simulink model "IEEE14_case"  (R2024b)
settings: Solver=FixedStepAuto  StartTime=0  StopTime=2  FixedStep=1e-7  RelTol=1e-3
values from neighbouring files (symbols this model uses):
  GFL_15_Bva = 0.009    [IEEE14_parameters.m]
  GFL_15_C_bus_pu = 7.179419    [IEEE14_parameters.m]
  GFL_15_f0 = 60    [IEEE14_parameters.m]
  GFL_15_I_id = 691.26967    [IEEE14_parameters.m]
  GFL_15_I_iq = 691.26967    [IEEE14_parameters.m]
  GFL_15_I_od = 45.2207    [IEEE14_parameters.m]
  GFL_15_I_oq = 45.2207    [IEEE14_parameters.m]
  GFL_15_I_pll = 0.78    [IEEE14_parameters.m]
  GFL_15_Kdi = 0.09    [IEEE14_parameters.m]
  GFL_15_Kdo = 0.9    [IEEE14_parameters.m]
  GFL_15_Kqi = 0.09    [IEEE14_parameters.m]
  GFL_15_Kqo = 0.9    [IEEE14_parameters.m]
  GFL_15_Lg_pu = 0.631447    [IEEE14_parameters.m]
  GFL_15_mode = 1    [IEEE14_parameters.m]
  GFL_15_P_id = 3.7166    [IEEE14_parameters.m]
  GFL_15_P_iq = 3.7166    [IEEE14_parameters.m]
  GFL_15_P_od = 0.4798    [IEEE14_parameters.m]
  GFL_15_P_oq = 0.4798    [IEEE14_parameters.m]
  GFL_15_P_pll = 290.42    [IEEE14_parameters.m]
  GFL_15_Qe_ref = 0.2    [IEEE14_parameters.m]
  GFL_15_Rg_pu = 0.024016    [IEEE14_parameters.m]
  GFL_15_Sbase = 1.000000e+4    (= 10000)    [IEEE14_parameters.m]
  GFL_15_Tdi = 0.01    [IEEE14_parameters.m]
  GFL_15_Tdo = 0.2    [IEEE14_parameters.m]
  GFL_15_Tqi = 0.01    [IEEE14_parameters.m]
  GFL_15_Tqo = 0.2    [IEEE14_parameters.m]
  GFL_15_Vbase = 380    [IEEE14_parameters.m]
  GFL_15_Vdc_ref = 1.011475    [IEEE14_parameters.m]
  GFL_15_Vdcbase = 700    [IEEE14_parameters.m]
  GFL_15_vq_ref = 0    [IEEE14_parameters.m]
  GFL_16_Bva = 0.002    [IEEE14_parameters.m]
  GFL_16_C_bus_pu = 7.179419    [IEEE14_parameters.m]
  GFL_16_f0 = 60    [IEEE14_parameters.m]
  GFL_16_I_id = 691.26967    [IEEE14_parameters.m]
  GFL_16_I_iq = 691.26967    [IEEE14_parameters.m]
  GFL_16_I_od = 45.2207    [IEEE14_parameters.m]
  GFL_16_I_oq = 45.2207    [IEEE14_parameters.m]
  GFL_16_I_pll = 0.78    [IEEE14_parameters.m]
  GFL_16_Kdi = 0.05    [IEEE14_parameters.m]
  GFL_16_Kdo = 0.5    [IEEE14_parameters.m]
  GFL_16_Kqi = 0.05    [IEEE14_parameters.m]
  GFL_16_Kqo = 0.5    [IEEE14_parameters.m]
  GFL_16_Lg_pu = 0.631447    [IEEE14_parameters.m]
  GFL_16_mode = 1    [IEEE14_parameters.m]
  GFL_16_P_id = 3.7166    [IEEE14_parameters.m]
  GFL_16_P_iq = 3.7166    [IEEE14_parameters.m]
  GFL_16_P_od = 0.4798    [IEEE14_parameters.m]
  GFL_16_P_oq = 0.4798    [IEEE14_parameters.m]
  GFL_16_P_pll = 290.42    [IEEE14_parameters.m]
  GFL_16_Qe_ref = 0.2    [IEEE14_parameters.m]
  GFL_16_Rg_pu = 0.024016    [IEEE14_parameters.m]
  GFL_16_Sbase = 1.000000e+4    (= 10000)    [IEEE14_parameters.m]
  GFL_16_Tdi = 0.01    [IEEE14_parameters.m]
  GFL_16_Tdo = 0.2    [IEEE14_parameters.m]
  GFL_16_Tqi = 0.01    [IEEE14_parameters.m]
  GFL_16_Tqo = 0.2    [IEEE14_parameters.m]
  GFL_16_Vbase = 380    [IEEE14_parameters.m]
  GFL_16_Vdc_ref = 1.01144    [IEEE14_parameters.m]
  GFL_16_Vdcbase = 700    [IEEE14_parameters.m]
  GFL_16_vq_ref = 0    [IEEE14_parameters.m]
  GFL_17_Bva = 0.002    [IEEE14_parameters.m]
  GFL_17_C_bus_pu = 7.179419    [IEEE14_parameters.m]
  GFL_17_f0 = 60    [IEEE14_parameters.m]
  GFL_17_I_id = 691.26967    [IEEE14_parameters.m]
  GFL_17_I_iq = 691.26967    [IEEE14_parameters.m]
  GFL_17_I_od = 45.2207    [IEEE14_parameters.m]
  GFL_17_I_oq = 45.2207    [IEEE14_parameters.m]
  GFL_17_I_pll = 0.78    [IEEE14_parameters.m]
  GFL_17_Kdi = 0.05    [IEEE14_parameters.m]
  GFL_17_Kdo = 0.5    [IEEE14_parameters.m]
  GFL_17_Kqi = 0.05    [IEEE14_parameters.m]
  GFL_17_Kqo = 0.5    [IEEE14_parameters.m]
  GFL_17_Lg_pu = 0.631447    [IEEE14_parameters.m]
  GFL_17_mode = 1    [IEEE14_parameters.m]
  GFL_17_P_id = 3.7166    [IEEE14_parameters.m]
  GFL_17_P_iq = 3.7166    [IEEE14_parameters.m]
  GFL_17_P_od = 0.4798    [IEEE14_parameters.m]
  GFL_17_P_oq = 0.4798    [IEEE14_parameters.m]
  GFL_17_P_pll = 290.42    [IEEE14_parameters.m]
  GFL_17_Qe_ref = 0.2    [IEEE14_parameters.m]
  GFL_17_Rg_pu = 0.024016    [IEEE14_parameters.m]
  GFL_17_Sbase = 1.000000e+4    (= 10000)    [IEEE14_parameters.m]
  GFL_17_Tdi = 0.01    [IEEE14_parameters.m]
  GFL_17_Tdo = 0.2    [IEEE14_parameters.m]
  GFL_17_Tqi = 0.01    [IEEE14_parameters.m]
  GFL_17_Tqo = 0.2    [IEEE14_parameters.m]
  GFL_17_Vbase = 380    [IEEE14_parameters.m]
  GFL_17_Vdc_ref = 1.011632    [IEEE14_parameters.m]
  GFL_17_Vdcbase = 700    [IEEE14_parameters.m]
  GFL_17_vq_ref = 0    [IEEE14_parameters.m]
  GFL_18_Bva = 0.002    [IEEE14_parameters.m]
  GFL_18_C_bus_pu = 7.179419    [IEEE14_parameters.m]
  GFL_18_f0 = 60    [IEEE14_parameters.m]
  GFL_18_I_id = 691.26967    [IEEE14_parameters.m]
  GFL_18_I_iq = 691.26967    [IEEE14_parameters.m]
  GFL_18_I_od = 45.2207    [IEEE14_parameters.m]
  GFL_18_I_oq = 45.2207    [IEEE14_parameters.m]
  GFL_18_I_pll = 0.78    [IEEE14_parameters.m]
  GFL_18_Kdi = 0.05    [IEEE14_parameters.m]
  GFL_18_Kdo = 0.5    [IEEE14_parameters.m]
  GFL_18_Kqi = 0.05    [IEEE14_parameters.m]
  GFL_18_Kqo = 0.5    [IEEE14_parameters.m]
  GFL_18_Lg_pu = 0.631447    [IEEE14_parameters.m]
  GFL_18_mode = 1    [IEEE14_parameters.m]
  GFL_18_P_id = 3.7166    [IEEE14_parameters.m]
  GFL_18_P_iq = 3.7166    [IEEE14_parameters.m]
  GFL_18_P_od = 0.4798    [IEEE14_parameters.m]
  GFL_18_P_oq = 0.4798    [IEEE14_parameters.m]
  GFL_18_P_pll = 290.42    [IEEE14_parameters.m]
  GFL_18_Qe_ref = 0.2    [IEEE14_parameters.m]
  GFL_18_Rg_pu = 0.024016    [IEEE14_parameters.m]
  GFL_18_Sbase = 1.000000e+4    (= 10000)    [IEEE14_parameters.m]
  GFL_18_Tdi = 0.01    [IEEE14_parameters.m]
  GFL_18_Tdo = 0.2    [IEEE14_parameters.m]
  GFL_18_Tqi = 0.01    [IEEE14_parameters.m]
  GFL_18_Tqo = 0.2    [IEEE14_parameters.m]
  GFL_18_Vbase = 380    [IEEE14_parameters.m]
  GFL_18_Vdc_ref = 1.011572    [IEEE14_parameters.m]
  GFL_18_Vdcbase = 700    [IEEE14_parameters.m]
  GFL_18_vq_ref = 0    [IEEE14_parameters.m]
  ... (+180 more)
(part 8 of 25)

== system IEEE14_case/AC_1/d_vq_bus_11_block ==
  note: d_vq_bus_11 in case14gfl
      | $9002.98797417909\,\mathrm{iq}_{\mathrm{bus},11}-376.991118430775\,\mathrm{vd}_{\mathrm{bus},11}$
      | Automatically generated on 2025-10-09 21:38:38 .
  Alge_iq_bus_11_f813e : Inport
  State_vd_bus_11_1dc97 : Inport  Port=2
  Constant_376.991118430775_261c0 : Constant  Value=376.991118430775
  Constant_9002.98797417909_ad544 : Constant  Value=9002.98797417909
  Product_24dc8 : Product
  Product_f14d9 : Product
  Subtract_a07b7 : Sum  Inputs=+-
  Blockout_d_vq_bus_11_d741b : Outport
  wires:
  Constant_9002.98797417909_ad544/1 -> Product_24dc8/1
  Alge_iq_bus_11_f813e/1 -> Product_24dc8/2
  Product_f14d9/1 -> Subtract_a07b7/2
  Constant_376.991118430775_261c0/1 -> Product_f14d9/1
  State_vd_bus_11_1dc97/1 -> Product_f14d9/2
  Product_24dc8/1 -> Subtract_a07b7/1
  Subtract_a07b7/1 -> Blockout_d_vq_bus_11_d741b/1

== system IEEE14_case/AC_1/d_vq_bus_12_block ==
  note: d_vq_bus_12 in case14gfl
      | $3672.44450708959\,\mathrm{iq}_{\mathrm{bus},12}-376.991118430775\,\mathrm{vd}_{\mathrm{bus},12}$
      | Automatically generated on 2025-10-09 21:38:40 .
  Alge_iq_bus_12_a824a : Inport
  State_vd_bus_12_1eb7a : Inport  Port=2
  Constant_3672.44450708959_5aba3 : Constant  Value=3672.44450708959
  Constant_376.991118430775_dbbc3 : Constant  Value=376.991118430775
  Product_f5227 : Product
  Product_ffd2a : Product
  Subtract_7b375 : Sum  Inputs=+-
  Blockout_d_vq_bus_12_08cfc : Outport
  wires:
  Subtract_7b375/1 -> Blockout_d_vq_bus_12_08cfc/1
  Constant_3672.44450708959_5aba3/1 -> Product_f5227/1
  State_vd_bus_12_1eb7a/1 -> Product_ffd2a/2
  Alge_iq_bus_12_a824a/1 -> Product_f5227/2
  Product_ffd2a/1 -> Subtract_7b375/2
  Constant_376.991118430775_dbbc3/1 -> Product_ffd2a/1
  Product_f5227/1 -> Subtract_7b375/1

== system IEEE14_case/AC_1/d_vq_bus_13_block ==
  note: d_vq_bus_13 in case14gfl
      | $2548.2341972351\,\mathrm{iq}_{\mathrm{bus},13}-376.991118430775\,\mathrm{vd}_{\mathrm{bus},13}$
      | Automatically generated on 2025-10-09 21:38:41 .
  Alge_iq_bus_13_d5ed4 : Inport
  State_vd_bus_13_68df6 : Inport  Port=2
  Constant_2548.2341972351_9e862 : Constant  Value=2548.2341972351
  Constant_376.991118430775_4e35a : Constant  Value=376.991118430775
  Product_0bf36 : Product
  Product_4bdfd : Product
  Subtract_14057 : Sum  Inputs=+-
  Blockout_d_vq_bus_13_eb8c6 : Outport
  wires:
  Subtract_14057/1 -> Blockout_d_vq_bus_13_eb8c6/1
  Constant_2548.2341972351_9e862/1 -> Product_0bf36/1
  Alge_iq_bus_13_d5ed4/1 -> Product_0bf36/2
  Constant_376.991118430775_4e35a/1 -> Product_4bdfd/1
  Product_0bf36/1 -> Subtract_14057/1
  State_vd_bus_13_68df6/1 -> Product_4bdfd/2
  Product_4bdfd/1 -> Subtract_14057/2

== system IEEE14_case/AC_1/d_vq_bus_14_block ==
  note: d_vq_bus_14 in case14gfl
      | $20061.7254996805\,\mathrm{iq}_{\mathrm{bus},14}-376.991118430775\,\mathrm{vd}_{\mathrm{bus},14}$
      | Automatically generated on 2025-10-09 21:38:43 .
  Alge_iq_bus_14_0b3bc : Inport
  State_vd_bus_14_b82c6 : Inport  Port=2
  Constant_20061.7254996805_caef0 : Constant  Value=20061.7254996805
  Constant_376.991118430775_d7d60 : Constant  Value=376.991118430775
  Product_cdac7 : Product
  Product_f9a80 : Product
  Subtract_506d5 : Sum  Inputs=+-
  Blockout_d_vq_bus_14_55ab8 : Outport
  wires:
  Constant_20061.7254996805_caef0/1 -> Product_f9a80/1
  Alge_iq_bus_14_0b3bc/1 -> Product_f9a80/2
  Product_cdac7/1 -> Subtract_506d5/2
  State_vd_bus_14_b82c6/1 -> Product_cdac7/2
  Constant_376.991118430775_d7d60/1 -> Product_cdac7/1
  Product_f9a80/1 -> Subtract_506d5/1
  Subtract_506d5/1 -> Blockout_d_vq_bus_14_55ab8/1

== system IEEE14_case/AC_1/d_vq_bus_15_block ==
  note: d_vq_bus_15 in case14gfl
      | $37699.1118430775\,\mathrm{iq}_{\mathrm{bus},15}-376.991118430775\,\mathrm{vd}_{\mathrm{bus},15}$
      | Automatically generated on 2025-10-09 21:38:44 .
  Alge_iq_bus_15_82ed5 : Inport
  State_vd_bus_15_ac75c : Inport  Port=2
  Constant_376.991118430775_eac41 : Constant  Value=376.991118430775
  Constant_37699.1118430775_013c4 : Constant  Value=37699.1118430775
  Product_6e790 : Product
  Product_7bd8f : Product
  Subtract_6bedb : Sum  Inputs=+-
  Blockout_d_vq_bus_15_3c6af : Outport
  wires:
  Constant_37699.1118430775_013c4/1 -> Product_7bd8f/1
  Product_6e790/1 -> Subtract_6bedb/2
  Constant_376.991118430775_eac41/1 -> Product_6e790/1
  Alge_iq_bus_15_82ed5/1 -> Product_7bd8f/2
  State_vd_bus_15_ac75c/1 -> Product_6e790/2
  Product_7bd8f/1 -> Subtract_6bedb/1
  Subtract_6bedb/1 -> Blockout_d_vq_bus_15_3c6af/1

== system IEEE14_case/AC_1/d_vq_bus_16_block ==
  note: d_vq_bus_16 in case14gfl
      | $37699.1118430775\,\mathrm{iq}_{\mathrm{bus},16}-376.991118430775\,\mathrm{vd}_{\mathrm{bus},16}$
      | Automatically generated on 2025-10-09 21:38:46 .
  Alge_iq_bus_16_45d99 : Inport
  State_vd_bus_16_358d8 : Inport  Port=2
  Constant_376.991118430775_caa10 : Constant  Value=376.991118430775
  Constant_37699.1118430775_2a605 : Constant  Value=37699.1118430775
  Product_3e245 : Product
  Product_65d14 : Product
  Subtract_b7523 : Sum  Inputs=+-
  Blockout_d_vq_bus_16_4b2eb : Outport
  wires:
  Alge_iq_bus_16_45d99/1 -> Product_65d14/2
  Constant_37699.1118430775_2a605/1 -> Product_65d14/1
  Product_3e245/1 -> Subtract_b7523/2
  Constant_376.991118430775_caa10/1 -> Product_3e245/1
  State_vd_bus_16_358d8/1 -> Product_3e245/2
  Product_65d14/1 -> Subtract_b7523/1
  Subtract_b7523/1 -> Blockout_d_vq_bus_16_4b2eb/1

== system IEEE14_case/AC_1/d_vq_bus_17_block ==
  note: d_vq_bus_17 in case14gfl
      | $37699.1118430775\,\mathrm{iq}_{\mathrm{bus},17}-376.991118430775\,\mathrm{vd}_{\mathrm{bus},17}$
      | Automatically generated on 2025-10-09 21:38:47 .
  Alge_iq_bus_17_e020e : Inport
  State_vd_bus_17_c4074 : Inport  Port=2
  Constant_376.991118430775_1fb98 : Constant  Value=376.991118430775
  Constant_37699.1118430775_26579 : Constant  Value=37699.1118430775
  Product_819ff : Product
  Product_cf9da : Product
  Subtract_66b2c : Sum  Inputs=+-
  Blockout_d_vq_bus_17_6d857 : Outport
  wires:
  Subtract_66b2c/1 -> Blockout_d_vq_bus_17_6d857/1
  Constant_37699.1118430775_26579/1 -> Product_cf9da/1
  Alge_iq_bus_17_e020e/1 -> Product_cf9da/2
  Constant_376.991118430775_1fb98/1 -> Product_819ff/1
  Product_cf9da/1 -> Subtract_66b2c/1
  State_vd_bus_17_c4074/1 -> Product_819ff/2
  Product_819ff/1 -> Subtract_66b2c/2

== system IEEE14_case/AC_1/d_vq_bus_18_block ==
  note: d_vq_bus_18 in case14gfl
      | $37699.1118430775\,\mathrm{iq}_{\mathrm{bus},18}-376.991118430775\,\mathrm{vd}_{\mathrm{bus},18}$
      | Automatically generated on 2025-10-09 21:38:49 .
  Alge_iq_bus_18_569e7 : Inport
  State_vd_bus_18_940ad : Inport  Port=2
  Constant_376.991118430775_f629c : Constant  Value=376.991118430775
  Constant_37699.1118430775_4526d : Constant  Value=37699.1118430775
  Product_ba63d : Product
  Product_f93d4 : Product
  Subtract_91363 : Sum  Inputs=+-
  Blockout_d_vq_bus_18_9e140 : Outport
  wires:
  Subtract_91363/1 -> Blockout_d_vq_bus_18_9e140/1
  Constant_37699.1118430775_4526d/1 -> Product_ba63d/1
  Alge_iq_bus_18_569e7/1 -> Product_ba63d/2
  Product_f93d4/1 -> Subtract_91363/2
  Constant_376.991118430775_f629c/1 -> Product_f93d4/1
  Product_ba63d/1 -> Subtract_91363/1
  State_vd_bus_18_940ad/1 -> Product_f93d4/2

== system IEEE14_case/AC_1/d_vq_bus_1_block ==
  note: d_vq_bus_1 in case14gfl
      | $7391.98271432892\,\mathrm{iq}_{\mathrm{bus},1}-376.991118430775\,\mathrm{vd}_{\mathrm{bus},1}$
      | Automatically generated on 2025-10-09 21:38:24 .
  Alge_iq_bus_1_7f6e6 : Inport
  State_vd_bus_1_cd54b : Inport  Port=2
  Constant_376.991118430775_bd390 : Constant  Value=376.991118430775
  Constant_7391.98271432892_c71cb : Constant  Value=7391.98271432892
  Product_b1b3b : Product
  Product_e1e81 : Product
  Subtract_afb98 : Sum  Inputs=+-
  Blockout_d_vq_bus_1_ae37f : Outport
  wires:
  Subtract_afb98/1 -> Blockout_d_vq_bus_1_ae37f/1
  Constant_7391.98271432892_c71cb/1 -> Product_e1e81/1
  Alge_iq_bus_1_7f6e6/1 -> Product_e1e81/2
  Constant_376.991118430775_bd390/1 -> Product_b1b3b/1
  Product_e1e81/1 -> Subtract_afb98/1
  State_vd_bus_1_cd54b/1 -> Product_b1b3b/2
  Product_b1b3b/1 -> Subtract_afb98/2

== system IEEE14_case/AC_1/d_vq_bus_2_block ==
  note: d_vq_bus_2 in case14gfl
      | $4564.05712385926\,\mathrm{iq}_{\mathrm{bus},2}-376.991118430775\,\mathrm{vd}_{\mathrm{bus},2}$
      | Automatically generated on 2025-10-09 21:38:25 .
  Alge_iq_bus_2_c94ee : Inport
  State_vd_bus_2_6d7a2 : Inport  Port=2
  Constant_376.991118430775_899fd : Constant  Value=376.991118430775
  Constant_4564.05712385926_bc465 : Constant  Value=4564.05712385926
  Product_17d0b : Product
  Product_9ea47 : Product
  Subtract_b4e59 : Sum  Inputs=+-
  Blockout_d_vq_bus_2_5ca2e : Outport
  wires:
  Subtract_b4e59/1 -> Blockout_d_vq_bus_2_5ca2e/1
  Constant_4564.05712385926_bc465/1 -> Product_9ea47/1
  Alge_iq_bus_2_c94ee/1 -> Product_9ea47/2
  Product_17d0b/1 -> Subtract_b4e59/2
  Constant_376.991118430775_899fd/1 -> Product_17d0b/1
  Product_9ea47/1 -> Subtract_b4e59/1
  State_vd_bus_2_6d7a2/1 -> Product_17d0b/2

== system IEEE14_case/AC_1/d_vq_bus_3_block ==
  note: d_vq_bus_3 in case14gfl
      | $13321.2409339497\,\mathrm{iq}_{\mathrm{bus},3}-376.991118430775\,\mathrm{vd}_{\mathrm{bus},3}$
      | Automatically generated on 2025-10-09 21:38:26 .
  Alge_iq_bus_3_8efd3 : Inport
  State_vd_bus_3_9f628 : Inport  Port=2
  Constant_13321.2409339497_e1066 : Constant  Value=13321.2409339497
  Constant_376.991118430775_27cd9 : Constant  Value=376.991118430775
  Product_520f1 : Product
  Product_bf7ac : Product
  Subtract_a0515 : Sum  Inputs=+-
  Blockout_d_vq_bus_3_9f56f : Outport
  wires:
  Constant_13321.2409339497_e1066/1 -> Product_bf7ac/1
  Alge_iq_bus_3_8efd3/1 -> Product_bf7ac/2
  Product_520f1/1 -> Subtract_a0515/2
  State_vd_bus_3_9f628/1 -> Product_520f1/2
  Constant_376.991118430775_27cd9/1 -> Product_520f1/1
  Product_bf7ac/1 -> Subtract_a0515/1
  Subtract_a0515/1 -> Blockout_d_vq_bus_3_9f56f/1

== system IEEE14_case/AC_1/d_vq_bus_4_block ==
  note: d_vq_bus_4 in case14gfl
      | $2583.02077551357\,\mathrm{iq}_{\mathrm{bus},4}-376.991118430775\,\mathrm{vd}_{\mathrm{bus},4}$
      | Automatically generated on 2025-10-09 21:38:28 .
  Alge_iq_bus_4_ff8e3 : Inport
  State_vd_bus_4_7baed : Inport  Port=2
  Constant_2583.02077551357_70067 : Constant  Value=2583.02077551357
  Constant_376.991118430775_0b7f7 : Constant  Value=376.991118430775
  Product_e62ad : Product
  Product_e77c5 : Product
  Subtract_93c34 : Sum  Inputs=+-
  Blockout_d_vq_bus_4_75eba : Outport
  wires:
  Constant_2583.02077551357_70067/1 -> Product_e62ad/1
  Product_e77c5/1 -> Subtract_93c34/2
  Constant_376.991118430775_0b7f7/1 -> Product_e77c5/1
  Alge_iq_bus_4_ff8e3/1 -> Product_e62ad/2
  State_vd_bus_4_7baed/1 -> Product_e77c5/2
  Product_e62ad/1 -> Subtract_93c34/1
  Subtract_93c34/1 -> Blockout_d_vq_bus_4_75eba/1

== system IEEE14_case/AC_1/d_vq_bus_5_block ==
  note: d_vq_bus_5 in case14gfl
      | $1402.86696243716\,\mathrm{iq}_{\mathrm{bus},5}-376.991118430775\,\mathrm{vd}_{\mathrm{bus},5}$
      | Automatically generated on 2025-10-09 21:38:29 .
  Alge_iq_bus_5_baf50 : Inport
  State_vd_bus_5_1cd26 : Inport  Port=2
  Constant_1402.86696243716_a548d : Constant  Value=1402.86696243716
  Constant_376.991118430775_949dd : Constant  Value=376.991118430775
  Product_29f51 : Product
  Product_fc59e : Product
  Subtract_c5361 : Sum  Inputs=+-
  Blockout_d_vq_bus_5_be7b6 : Outport
  wires:
  Alge_iq_bus_5_baf50/1 -> Product_fc59e/2
  Constant_1402.86696243716_a548d/1 -> Product_fc59e/1
  Constant_376.991118430775_949dd/1 -> Product_29f51/1
  State_vd_bus_5_1cd26/1 -> Product_29f51/2
  Product_fc59e/1 -> Subtract_c5361/1
  Product_29f51/1 -> Subtract_c5361/2
  Subtract_c5361/1 -> Blockout_d_vq_bus_5_be7b6/1

== system IEEE14_case/AC_1/d_vq_bus_6_block ==
  note: d_vq_bus_6 in case14gfl
      | $1302.18631108196\,\mathrm{iq}_{\mathrm{bus},6}-376.991118430775\,\mathrm{vd}_{\mathrm{bus},6}$
      | Automatically generated on 2025-10-09 21:38:31 .
  Alge_iq_bus_6_86836 : Inport
  State_vd_bus_6_d464c : Inport  Port=2
  Constant_1302.18631108196_07ceb : Constant  Value=1302.18631108196
  Constant_376.991118430775_01266 : Constant  Value=376.991118430775
  Product_34f15 : Product
  Product_6915d : Product
  Subtract_2b736 : Sum  Inputs=+-
  Blockout_d_vq_bus_6_55bf0 : Outport
  wires:
  Subtract_2b736/1 -> Blockout_d_vq_bus_6_55bf0/1
  Constant_1302.18631108196_07ceb/1 -> Product_34f15/1
  Alge_iq_bus_6_86836/1 -> Product_34f15/2
  Product_6915d/1 -> Subtract_2b736/2
  Constant_376.991118430775_01266/1 -> Product_6915d/1
  Product_34f15/1 -> Subtract_2b736/1
  State_vd_bus_6_d464c/1 -> Product_6915d/2

== system IEEE14_case/AC_1/d_vq_bus_7_block ==
  note: d_vq_bus_7 in case14gfl
      | $3504.63555759756\,\mathrm{iq}_{\mathrm{bus},7}-376.991118430775\,\mathrm{vd}_{\mathrm{bus},7}$
      | Automatically generated on 2025-10-09 21:38:32 .
  Alge_iq_bus_7_36c94 : Inport
  State_vd_bus_7_1c88a : Inport  Port=2
  Constant_3504.63555759756_fabdc : Constant  Value=3504.63555759756
  Constant_376.991118430775_640aa : Constant  Value=376.991118430775
  Product_9d0b8 : Product
  Product_d63cb : Product
  Subtract_76f89 : Sum  Inputs=+-
  Blockout_d_vq_bus_7_86357 : Outport
  wires:
  Constant_3504.63555759756_fabdc/1 -> Product_d63cb/1
  Alge_iq_bus_7_36c94/1 -> Product_d63cb/2
  Product_9d0b8/1 -> Subtract_76f89/2
  Constant_376.991118430775_640aa/1 -> Product_9d0b8/1
  State_vd_bus_7_1c88a/1 -> Product_9d0b8/2
  Product_d63cb/1 -> Subtract_76f89/1
  Subtract_76f89/1 -> Blockout_d_vq_bus_7_86357/1

== system IEEE14_case/AC_1/d_vq_bus_8_block ==
  note: d_vq_bus_8 in case14gfl
      | $2490.79058651093\,\mathrm{iq}_{\mathrm{bus},8}-376.991118430775\,\mathrm{vd}_{\mathrm{bus},8}$
      | Automatically generated on 2025-10-09 21:38:34 .
  Alge_iq_bus_8_97cc9 : Inport
  State_vd_bus_8_3801a : Inport  Port=2
  Constant_2490.79058651093_f1201 : Constant  Value=2490.79058651093
  Constant_376.991118430775_4ed82 : Constant  Value=376.991118430775
  Product_0f968 : Product
  Product_ef9ef : Product
  Subtract_8ea8e : Sum  Inputs=+-
  Blockout_d_vq_bus_8_795e4 : Outport
  wires:
  Subtract_8ea8e/1 -> Blockout_d_vq_bus_8_795e4/1
  Constant_2490.79058651093_f1201/1 -> Product_ef9ef/1
  Alge_iq_bus_8_97cc9/1 -> Product_ef9ef/2
  Product_0f968/1 -> Subtract_8ea8e/2
  Constant_376.991118430775_4ed82/1 -> Product_0f968/1
  Product_ef9ef/1 -> Subtract_8ea8e/1
  State_vd_bus_8_3801a/1 -> Product_0f968/2

== system IEEE14_case/AC_1/d_vq_bus_9_block ==
  note: d_vq_bus_9 in case14gfl
      | $1523.0703691556\,\mathrm{iq}_{\mathrm{bus},9}-376.991118430775\,\mathrm{vd}_{\mathrm{bus},9}$
      | Automatically generated on 2025-10-09 21:38:35 .
  Alge_iq_bus_9_5db18 : Inport
  State_vd_bus_9_ab45c : Inport  Port=2
  Constant_1523.0703691556_10aef : Constant  Value=1523.0703691556
  Constant_376.991118430775_97651 : Constant  Value=376.991118430775
  Product_200ef : Product
  Product_6bff3 : Product
  Subtract_8eb2d : Sum  Inputs=+-
  Blockout_d_vq_bus_9_d5b49 : Outport
  wires:
  Constant_1523.0703691556_10aef/1 -> Product_6bff3/1
  Constant_376.991118430775_97651/1 -> Product_200ef/1
  Alge_iq_bus_9_5db18/1 -> Product_6bff3/2
  Product_200ef/1 -> Subtract_8eb2d/2
  State_vd_bus_9_ab45c/1 -> Product_200ef/2
  Product_6bff3/1 -> Subtract_8eb2d/1
  Subtract_8eb2d/1 -> Blockout_d_vq_bus_9_d5b49/1

== system IEEE14_case/AC_1/id_bus_10_block ==
  note: id_bus_10 in case14gfl
      | $\mathrm{id}_{\mathrm{line},9,10}-\mathrm{id}_{\mathrm{load},10}-\mathrm{id}_{\mathrm{line},10,11}$
      | Automatically generated on 2025-10-09 21:40:23 .
  State_id_load_10_5dfe0 : Inport
  State_id_line_9_10_2483c : Inport  Port=2
  State_id_line_10_11_6295b : Inport  Port=3
  Add_b3e74 : Sum
  Constant_-1_7254c : Constant  Value=-1
  Product_2a7e4 : Product
  Subtract_4a90e : Sum  Inputs=+-
  Blockout_id_bus_10_ed934 : Outport
  wires:
  State_id_line_9_10_2483c/1 -> Add_b3e74/2
  Constant_-1_7254c/1 -> Product_2a7e4/1
  Add_b3e74/1 -> Subtract_4a90e/1
  Product_2a7e4/1 -> Add_b3e74/1
  State_id_load_10_5dfe0/1 -> Product_2a7e4/2
  Subtract_4a90e/1 -> Blockout_id_bus_10_ed934/1
  State_id_line_10_11_6295b/1 -> Subtract_4a90e/2

== system IEEE14_case/AC_1/id_bus_11_block ==
  note: id_bus_11 in case14gfl
      | $\mathrm{id}_{\mathrm{line},6,11}-\mathrm{id}_{\mathrm{load},11}+\mathrm{id}_{\mathrm{line},10,11}-\mathrm{id}_{\mathrm{line},11,15}$
      | Automatically generated on 2025-10-09 21:40:24 .
  State_id_load_11_85329 : Inport
  State_id_line_6_11_4f772 : Inport  Port=2
  State_id_line_10_11_3f962 : Inport  Port=3
  State_id_line_11_15_2f637 : Inport  Port=4
  Add_487b5 : Sum
  Add_caf04 : Sum
  Constant_-1_8d3ad : Constant  Value=-1
  Product_7a38a : Product
  Subtract_db9fd : Sum  Inputs=+-
  Blockout_id_bus_11_f1534 : Outport
  wires:
  Constant_-1_8d3ad/1 -> Product_7a38a/1
  Product_7a38a/1 -> Add_487b5/1
  Add_487b5/1 -> Add_caf04/1
  State_id_line_6_11_4f772/1 -> Add_487b5/2
  State_id_load_11_85329/1 -> Product_7a38a/2
  State_id_line_10_11_3f962/1 -> Add_caf04/2
  Add_caf04/1 -> Subtract_db9fd/1
  State_id_line_11_15_2f637/1 -> Subtract_db9fd/2
  Subtract_db9fd/1 -> Blockout_id_bus_11_f1534/1

== system IEEE14_case/AC_1/id_bus_12_block ==
  note: id_bus_12 in case14gfl
      | $\mathrm{id}_{\mathrm{line},6,12}-\mathrm{id}_{\mathrm{load},12}-\mathrm{id}_{\mathrm{line},12,13}-\mathrm{id}_{\mathrm{line},12,16}$
      | Automatically generated on 2025-10-09 21:40:26 .
  State_id_load_12_a6028 : Inport
  State_id_line_6_12_49cbb : Inport  Port=2
  State_id_line_12_13_b0c21 : Inport  Port=3
  State_id_line_12_16_716c0 : Inport  Port=4
  Add_6264a : Sum
  Constant_-1_16dc0 : Constant  Value=-1
  Product_a23ec : Product
  Subtract_5bbcc : Sum  Inputs=+-
  Subtract_e4954 : Sum  Inputs=+-
  Blockout_id_bus_12_1147b : Outport
  wires:
  State_id_line_12_16_716c0/1 -> Subtract_5bbcc/2
  Constant_-1_16dc0/1 -> Product_a23ec/1
  Product_a23ec/1 -> Add_6264a/1
  Add_6264a/1 -> Subtract_e4954/1
  State_id_line_6_12_49cbb/1 -> Add_6264a/2
  State_id_load_12_a6028/1 -> Product_a23ec/2
  State_id_line_12_13_b0c21/1 -> Subtract_e4954/2
  Subtract_e4954/1 -> Subtract_5bbcc/1
  Subtract_5bbcc/1 -> Blockout_id_bus_12_1147b/1

== system IEEE14_case/AC_1/id_bus_13_block ==
  note: id_bus_13 in case14gfl
      | $\mathrm{id}_{\mathrm{line},6,13}-\mathrm{id}_{\mathrm{load},13}+\mathrm{id}_{\mathrm{line},12,13}-\mathrm{id}_{\mathrm{line},13,14}-\mathrm{id}_{\mathrm{line},13,17}$
      | Automatically generated on 2025-10-09 21:40:28 .
  State_id_load_13_0fa38 : Inport
  State_id_line_6_13_33910 : Inport  Port=2
  State_id_line_12_13_8b355 : Inport  Port=3
  State_id_line_13_14_d0ea7 : Inport  Port=4
  State_id_line_13_17_1d2fa : Inport  Port=5
  Add_b4b15 : Sum
  Add_d7b27 : Sum
  Constant_-1_73811 : Constant  Value=-1
  Product_b982f : Product
  Subtract_41210 : Sum  Inputs=+-
  Subtract_cbe59 : Sum  Inputs=+-
  Blockout_id_bus_13_73688 : Outport
  wires:
  Constant_-1_73811/1 -> Product_b982f/1
  Product_b982f/1 -> Add_b4b15/1
  State_id_load_13_0fa38/1 -> Product_b982f/2
  State_id_line_12_13_8b355/1 -> Add_d7b27/2
  State_id_line_6_13_33910/1 -> Add_b4b15/2
  Add_b4b15/1 -> Add_d7b27/1
  Add_d7b27/1 -> Subtract_cbe59/1
  State_id_line_13_14_d0ea7/1 -> Subtract_cbe59/2
  Subtract_cbe59/1 -> Subtract_41210/1
  State_id_line_13_17_1d2fa/1 -> Subtract_41210/2
  Subtract_41210/1 -> Blockout_id_bus_13_73688/1

== system IEEE14_case/AC_1/id_bus_14_block ==
  note: id_bus_14 in case14gfl
      | $\mathrm{id}_{\mathrm{line},9,14}-\mathrm{id}_{\mathrm{load},14}+\mathrm{id}_{\mathrm{line},13,14}-\mathrm{id}_{\mathrm{line},14,18}$
      | Automatically generated on 2025-10-09 21:40:30 .
  State_id_load_14_1cf8a : Inport
  State_id_line_9_14_3a619 : Inport  Port=2
  State_id_line_13_14_e8dab : Inport  Port=3
  State_id_line_14_18_ae0a4 : Inport  Port=4
  Add_0909d : Sum
  Add_8825a : Sum
  Constant_-1_2a839 : Constant  Value=-1
  Product_6b33f : Product
  Subtract_d2b6f : Sum  Inputs=+-
  Blockout_id_bus_14_6847e : Outport
  wires:
  Add_0909d/1 -> Subtract_d2b6f/1
  State_id_line_13_14_e8dab/1 -> Add_0909d/2
  Subtract_d2b6f/1 -> Blockout_id_bus_14_6847e/1
  State_id_line_9_14_3a619/1 -> Add_8825a/2
  Constant_-1_2a839/1 -> Product_6b33f/1
  State_id_load_14_1cf8a/1 -> Product_6b33f/2
  State_id_line_14_18_ae0a4/1 -> Subtract_d2b6f/2
  Product_6b33f/1 -> Add_8825a/1
  Add_8825a/1 -> Add_0909d/1

== system IEEE14_case/AC_1/id_bus_15_block ==
  note: id_bus_15 in case14gfl
      | $\mathrm{id}_{\mathrm{GFL},15}+\mathrm{id}_{\mathrm{line},11,15}$
      | Automatically generated on 2025-10-09 21:40:33 .
  Input_id_GFL_15_c7559 : Inport
  State_id_line_11_15_010a9 : Inport  Port=2
  Add_2ecf8 : Sum
  Blockout_id_bus_15_e9971 : Outport
  wires:
  State_id_line_11_15_010a9/1 -> Add_2ecf8/2
  Input_id_GFL_15_c7559/1 -> Add_2ecf8/1
  Add_2ecf8/1 -> Blockout_id_bus_15_e9971/1

== system IEEE14_case/AC_1/id_bus_16_block ==
  note: id_bus_16 in case14gfl
      | $\mathrm{id}_{\mathrm{GFL},16}+\mathrm{id}_{\mathrm{line},12,16}$
      | Automatically generated on 2025-10-09 21:40:36 .
  Input_id_GFL_16_67778 : Inport
  State_id_line_12_16_7c95c : Inport  Port=2
  Add_9dc53 : Sum
  Blockout_id_bus_16_bdc3f : Outport
  wires:
  State_id_line_12_16_7c95c/1 -> Add_9dc53/2
  Input_id_GFL_16_67778/1 -> Add_9dc53/1
  Add_9dc53/1 -> Blockout_id_bus_16_bdc3f/1

== system IEEE14_case/AC_1/id_bus_17_block ==
  note: id_bus_17 in case14gfl
      | $\mathrm{id}_{\mathrm{GFL},17}+\mathrm{id}_{\mathrm{line},13,17}$
      | Automatically generated on 2025-10-09 21:40:38 .
  Input_id_GFL_17_1404c : Inport
  State_id_line_13_17_58c1b : Inport  Port=2
  Add_d53d4 : Sum
  Blockout_id_bus_17_789d1 : Outport
  wires:
  State_id_line_13_17_58c1b/1 -> Add_d53d4/2
  Input_id_GFL_17_1404c/1 -> Add_d53d4/1
  Add_d53d4/1 -> Blockout_id_bus_17_789d1/1

== system IEEE14_case/AC_1/id_bus_18_block ==
  note: id_bus_18 in case14gfl
      | $\mathrm{id}_{\mathrm{GFL},18}+\mathrm{id}_{\mathrm{line},14,18}$
      | Automatically generated on 2025-10-09 21:40:41 .
  Input_id_GFL_18_1db57 : Inport
  State_id_line_14_18_0ac94 : Inport  Port=2
  Add_4feb4 : Sum
  Blockout_id_bus_18_37cb9 : Outport
  wires:
  State_id_line_14_18_0ac94/1 -> Add_4feb4/2
  Input_id_GFL_18_1db57/1 -> Add_4feb4/1
  Add_4feb4/1 -> Blockout_id_bus_18_37cb9/1

== system IEEE14_case/AC_1/id_bus_1_block ==
  note: id_bus_1 in case14gfl
      | $\mathrm{id}_{\mathrm{SG},D,1}-\mathrm{id}_{\mathrm{line},1,2}-\mathrm{id}_{\mathrm{line},1,5}$
      | Automatically generated on 2025-10-09 21:40:03 .
  Input_id_SG_D_1_3327d : Inport
  State_id_line_1_2_9da7e : Inport  Port=2
  State_id_line_1_5_b6c3a : Inport  Port=3
  Subtract_bdc4f : Sum  Inputs=+-
  Subtract_f2024 : Sum  Inputs=+-
  Blockout_id_bus_1_ba05b : Outport
  wires:
  State_id_line_1_5_b6c3a/1 -> Subtract_f2024/2
  Input_id_SG_D_1_3327d/1 -> Subtract_bdc4f/1
  State_id_line_1_2_9da7e/1 -> Subtract_bdc4f/2
  Subtract_bdc4f/1 -> Subtract_f2024/1
  Subtract_f2024/1 -> Blockout_id_bus_1_ba05b/1

== system IEEE14_case/AC_1/id_bus_2_block ==
  note: id_bus_2 in case14gfl
      | $\mathrm{id}_{\mathrm{SG},D,2}-\mathrm{id}_{\mathrm{load},2}+\mathrm{id}_{\mathrm{line},1,2}-\mathrm{id}_{\mathrm{line},2,3}-\mathrm{id}_{\mathrm{line},2,4}-\mathrm{id}_{\mathrm{line},2,5}$
      | Automatically generated on 2025-10-09 21:40:06 .
  Input_id_SG_D_2_87b72 : Inport
  State_id_load_2_24351 : Inport  Port=2
  State_id_line_1_2_672bc : Inport  Port=3
  State_id_line_2_3_47528 : Inport  Port=4
  State_id_line_2_4_54727 : Inport  Port=5
  State_id_line_2_5_398b7 : Inport  Port=6
  Add_d3f46 : Sum
  Subtract_03279 : Sum  Inputs=+-
  Subtract_6b1c4 : Sum  Inputs=+-
  Subtract_aa1a1 : Sum  Inputs=+-
  Subtract_ec35f : Sum  Inputs=+-
  Blockout_id_bus_2_89082 : Outport
  wires:
  Input_id_SG_D_2_87b72/1 -> Subtract_03279/1
  Subtract_03279/1 -> Add_d3f46/1
  Add_d3f46/1 -> Subtract_aa1a1/1
  State_id_line_1_2_672bc/1 -> Add_d3f46/2
  State_id_load_2_24351/1 -> Subtract_03279/2
  State_id_line_2_3_47528/1 -> Subtract_aa1a1/2
  Subtract_aa1a1/1 -> Subtract_ec35f/1
  State_id_line_2_4_54727/1 -> Subtract_ec35f/2
  Subtract_ec35f/1 -> Subtract_6b1c4/1
  State_id_line_2_5_398b7/1 -> Subtract_6b1c4/2
  Subtract_6b1c4/1 -> Blockout_id_bus_2_89082/1

== system IEEE14_case/AC_1/id_bus_3_block ==
  note: id_bus_3 in case14gfl
      | $\mathrm{id}_{\mathrm{SG},D,3}-\mathrm{id}_{\mathrm{load},3}+\mathrm{id}_{\mathrm{line},2,3}-\mathrm{id}_{\mathrm{line},3,4}$
      | Automatically generated on 2025-10-09 21:40:08 .
  Input_id_SG_D_3_ffe04 : Inport
  State_id_load_3_b4943 : Inport  Port=2
  State_id_line_2_3_0c1e5 : Inport  Port=3
  State_id_line_3_4_0527c : Inport  Port=4
  Add_a702f : Sum
  Subtract_83a75 : Sum  Inputs=+-
  Subtract_c699a : Sum  Inputs=+-
  Blockout_id_bus_3_cecd1 : Outport
  wires:
  Subtract_83a75/1 -> Blockout_id_bus_3_cecd1/1
  Subtract_c699a/1 -> Add_a702f/1
  Input_id_SG_D_3_ffe04/1 -> Subtract_c699a/1
  Add_a702f/1 -> Subtract_83a75/1
  State_id_line_2_3_0c1e5/1 -> Add_a702f/2
  State_id_load_3_b4943/1 -> Subtract_c699a/2
  State_id_line_3_4_0527c/1 -> Subtract_83a75/2

== system IEEE14_case/AC_1/id_bus_4_block ==
  note: id_bus_4 in case14gfl
      | $\mathrm{id}_{\mathrm{line},2,4}-\mathrm{id}_{\mathrm{load},4}+\mathrm{id}_{\mathrm{line},3,4}-\mathrm{id}_{\mathrm{line},4,5}-\mathrm{id}_{\mathrm{line},4,7}-\mathrm{id}_{\mathrm{line},4,9}$
      | Automatically generated on 2025-10-09 21:40:10 .
  State_id_load_4_4d084 : Inport
  State_id_line_2_4_71476 : Inport  Port=2
  State_id_line_3_4_6920e : Inport  Port=3
  State_id_line_4_5_4eaac : Inport  Port=4
  State_id_line_4_7_02fe7 : Inport  Port=5
  State_id_line_4_9_61110 : Inport  Port=6
  Add_b90e8 : Sum
  Add_d07e9 : Sum
  Constant_-1_6e42c : Constant  Value=-1
  Product_e3529 : Product
  Subtract_88d6a : Sum  Inputs=+-
  Subtract_a273d : Sum  Inputs=+-
  Subtract_b185a : Sum  Inputs=+-
  Blockout_id_bus_4_5067c : Outport
  wires:
  State_id_line_3_4_6920e/1 -> Add_d07e9/2
  State_id_line_2_4_71476/1 -> Add_b90e8/2
  Constant_-1_6e42c/1 -> Product_e3529/1
  Product_e3529/1 -> Add_b90e8/1
  State_id_load_4_4d084/1 -> Product_e3529/2
  Add_b90e8/1 -> Add_d07e9/1
  Add_d07e9/1 -> Subtract_b185a/1
  State_id_line_4_5_4eaac/1 -> Subtract_b185a/2
  Subtract_b185a/1 -> Subtract_88d6a/1
  State_id_line_4_7_02fe7/1 -> Subtract_88d6a/2
  Subtract_88d6a/1 -> Subtract_a273d/1
  State_id_line_4_9_61110/1 -> Subtract_a273d/2
  Subtract_a273d/1 -> Blockout_id_bus_4_5067c/1

== system IEEE14_case/AC_1/id_bus_5_block ==
  note: id_bus_5 in case14gfl
      | $\mathrm{id}_{\mathrm{line},1,5}-\mathrm{id}_{\mathrm{load},5}+\mathrm{id}_{\mathrm{line},2,5}+\mathrm{id}_{\mathrm{line},4,5}-\mathrm{id}_{\mathrm{line},5,6}$
      | Automatically generated on 2025-10-09 21:40:12 .
  State_id_load_5_1b867 : Inport
  State_id_line_1_5_464f3 : Inport  Port=2
  State_id_line_2_5_8adac : Inport  Port=3
  State_id_line_4_5_5de68 : Inport  Port=4
  State_id_line_5_6_d193e : Inport  Port=5
  Add_a6bd2 : Sum
  Add_ad556 : Sum
  Add_ea241 : Sum
  Constant_-1_43326 : Constant  Value=-1
  Product_bc7f8 : Product
  Subtract_cc0f7 : Sum  Inputs=+-
  Blockout_id_bus_5_9fe33 : Outport
  wires:
  Constant_-1_43326/1 -> Product_bc7f8/1
  Product_bc7f8/1 -> Add_a6bd2/1
  Add_ea241/1 -> Subtract_cc0f7/1
  Add_a6bd2/1 -> Add_ad556/1
  State_id_load_5_1b867/1 -> Product_bc7f8/2
  State_id_line_2_5_8adac/1 -> Add_ad556/2
  State_id_line_1_5_464f3/1 -> Add_a6bd2/2
  Add_ad556/1 -> Add_ea241/1
  State_id_line_4_5_5de68/1 -> Add_ea241/2
  State_id_line_5_6_d193e/1 -> Subtract_cc0f7/2
  Subtract_cc0f7/1 -> Blockout_id_bus_5_9fe33/1

== system IEEE14_case/AC_1/id_bus_6_block ==
  note: id_bus_6 in case14gfl
      | $\mathrm{id}_{\mathrm{SG},D,6}-\mathrm{id}_{\mathrm{load},6}+\mathrm{id}_{\mathrm{line},5,6}-\mathrm{id}_{\mathrm{line},6,11}-\mathrm{id}_{\mathrm{line},6,12}-\mathrm{id}_{\mathrm{line},6,13}$
      | Automatically generated on 2025-10-09 21:40:15 .
  Input_id_SG_D_6_e5cad : Inport
  State_id_load_6_c7fc2 : Inport  Port=2
  State_id_line_5_6_cecb9 : Inport  Port=3
  State_id_line_6_11_01f81 : Inport  Port=4
  State_id_line_6_12_d416e : Inport  Port=5
  State_id_line_6_13_76e25 : Inport  Port=6
  Add_bcbea : Sum
  Subtract_541e7 : Sum  Inputs=+-
  Subtract_58720 : Sum  Inputs=+-
  Subtract_9b426 : Sum  Inputs=+-
  Subtract_c06a4 : Sum  Inputs=+-
  Blockout_id_bus_6_5cca2 : Outport
  wires:
  Input_id_SG_D_6_e5cad/1 -> Subtract_58720/1
  Subtract_58720/1 -> Add_bcbea/1
  Add_bcbea/1 -> Subtract_9b426/1
  State_id_load_6_c7fc2/1 -> Subtract_58720/2
  State_id_line_6_11_01f81/1 -> Subtract_9b426/2
  State_id_line_5_6_cecb9/1 -> Add_bcbea/2
  Subtract_9b426/1 -> Subtract_541e7/1
  State_id_line_6_12_d416e/1 -> Subtract_541e7/2
  Subtract_541e7/1 -> Subtract_c06a4/1
  State_id_line_6_13_76e25/1 -> Subtract_c06a4/2
  Subtract_c06a4/1 -> Blockout_id_bus_6_5cca2/1

== system IEEE14_case/AC_1/id_bus_7_block ==
  note: id_bus_7 in case14gfl
      | $\mathrm{id}_{\mathrm{line},4,7}-\mathrm{id}_{\mathrm{line},7,8}-\mathrm{id}_{\mathrm{line},7,9}$
      | Automatically generated on 2025-10-09 21:40:17 .
  State_id_line_4_7_887cf : Inport
  State_id_line_7_8_a9fc4 : Inport  Port=2
  State_id_line_7_9_11a60 : Inport  Port=3
  Subtract_12466 : Sum  Inputs=+-
  Subtract_34946 : Sum  Inputs=+-
  Blockout_id_bus_7_ec462 : Outport
  wires:
  State_id_line_4_7_887cf/1 -> Subtract_12466/1
  State_id_line_7_8_a9fc4/1 -> Subtract_12466/2
  Subtract_34946/1 -> Blockout_id_bus_7_ec462/1
  Subtract_12466/1 -> Subtract_34946/1
  State_id_line_7_9_11a60/1 -> Subtract_34946/2

== system IEEE14_case/AC_1/id_bus_8_block ==
  note: id_bus_8 in case14gfl
      | $\mathrm{id}_{\mathrm{SG},D,8}+\mathrm{id}_{\mathrm{line},7,8}$
      | Automatically generated on 2025-10-09 21:40:19 .
  Input_id_SG_D_8_15cec : Inport
  State_id_line_7_8_1f3e4 : Inport  Port=2
  Add_9a4b3 : Sum
  Blockout_id_bus_8_d2e4f : Outport
  wires:
  Add_9a4b3/1 -> Blockout_id_bus_8_d2e4f/1
  Input_id_SG_D_8_15cec/1 -> Add_9a4b3/1
  State_id_line_7_8_1f3e4/1 -> Add_9a4b3/2

== system IEEE14_case/AC_1/id_bus_9_block ==
  note: id_bus_9 in case14gfl
      | $\mathrm{id}_{\mathrm{line},4,9}-\mathrm{id}_{\mathrm{load},9}+\mathrm{id}_{\mathrm{line},7,9}-\mathrm{id}_{\mathrm{line},9,10}-\mathrm{id}_{\mathrm{line},9,14}$
      | Automatically generated on 2025-10-09 21:40:21 .
  State_id_load_9_3577c : Inport
  State_id_line_4_9_8b9da : Inport  Port=2
  State_id_line_7_9_16065 : Inport  Port=3
  State_id_line_9_10_faf7e : Inport  Port=4
  State_id_line_9_14_00d21 : Inport  Port=5
  Add_0a8d4 : Sum
  Add_56e96 : Sum
  Constant_-1_1728c : Constant  Value=-1
  Product_b19ef : Product
  Subtract_891af : Sum  Inputs=+-
  Subtract_bdce0 : Sum  Inputs=+-
  Blockout_id_bus_9_1c066 : Outport
  wires:
  Subtract_891af/1 -> Blockout_id_bus_9_1c066/1
  Subtract_bdce0/1 -> Subtract_891af/1
  State_id_line_7_9_16065/1 -> Add_56e96/2
  State_id_line_4_9_8b9da/1 -> Add_0a8d4/2
  Constant_-1_1728c/1 -> Product_b19ef/1
  Product_b19ef/1 -> Add_0a8d4/1
  State_id_load_9_3577c/1 -> Product_b19ef/2
  Add_0a8d4/1 -> Add_56e96/1
  Add_56e96/1 -> Subtract_bdce0/1
  State_id_line_9_10_faf7e/1 -> Subtract_bdce0/2
  State_id_line_9_14_00d21/1 -> Subtract_891af/2

== system IEEE14_case/AC_1/iq_bus_10_block ==
  note: iq_bus_10 in case14gfl
      | $\mathrm{iq}_{\mathrm{line},9,10}-\mathrm{iq}_{\mathrm{load},10}-\mathrm{iq}_{\mathrm{line},10,11}$
      | Automatically generated on 2025-10-09 21:40:23 .
  State_iq_load_10_2ce70 : Inport
  State_iq_line_9_10_4cded : Inport  Port=2
  State_iq_line_10_11_32883 : Inport  Port=3
  Add_51095 : Sum
  Constant_-1_0a19e : Constant  Value=-1
  Product_e9f60 : Product
  Subtract_b173d : Sum  Inputs=+-
  Blockout_iq_bus_10_4d9cc : Outport
  wires:
  Add_51095/1 -> Subtract_b173d/1
  Product_e9f60/1 -> Add_51095/1
  Constant_-1_0a19e/1 -> Product_e9f60/1
  State_iq_line_9_10_4cded/1 -> Add_51095/2
  State_iq_load_10_2ce70/1 -> Product_e9f60/2
  State_iq_line_10_11_32883/1 -> Subtract_b173d/2
  Subtract_b173d/1 -> Blockout_iq_bus_10_4d9cc/1

== system IEEE14_case/AC_1/iq_bus_11_block ==
  note: iq_bus_11 in case14gfl
      | $\mathrm{iq}_{\mathrm{line},6,11}-\mathrm{iq}_{\mathrm{load},11}+\mathrm{iq}_{\mathrm{line},10,11}-\mathrm{iq}_{\mathrm{line},11,15}$
      | Automatically generated on 2025-10-09 21:40:25 .
  State_iq_load_11_c9523 : Inport
  State_iq_line_6_11_3bc55 : Inport  Port=2
  State_iq_line_10_11_5b2aa : Inport  Port=3
  State_iq_line_11_15_05d46 : Inport  Port=4
  Add_0662d : Sum
  Add_98c18 : Sum
  Constant_-1_8e433 : Constant  Value=-1
  Product_f2178 : Product
  Subtract_ed55f : Sum  Inputs=+-
  Blockout_iq_bus_11_5f78a : Outport
  wires:
  Constant_-1_8e433/1 -> Product_f2178/1
  Product_f2178/1 -> Add_0662d/1
  State_iq_load_11_c9523/1 -> Product_f2178/2
  State_iq_line_10_11_5b2aa/1 -> Add_98c18/2
  State_iq_line_6_11_3bc55/1 -> Add_0662d/2
  Add_0662d/1 -> Add_98c18/1
  Add_98c18/1 -> Subtract_ed55f/1
  State_iq_line_11_15_05d46/1 -> Subtract_ed55f/2
  Subtract_ed55f/1 -> Blockout_iq_bus_11_5f78a/1

== system IEEE14_case/AC_1/iq_bus_12_block ==
  note: iq_bus_12 in case14gfl
      | $\mathrm{iq}_{\mathrm{line},6,12}-\mathrm{iq}_{\mathrm{load},12}-\mathrm{iq}_{\mathrm{line},12,13}-\mathrm{iq}_{\mathrm{line},12,16}$
      | Automatically generated on 2025-10-09 21:40:27 .
  State_iq_load_12_82e1a : Inport
  State_iq_line_6_12_a1863 : Inport  Port=2
  State_iq_line_12_13_b5bd7 : Inport  Port=3
  State_iq_line_12_16_8cacc : Inport  Port=4
  Add_e4c6d : Sum
  Constant_-1_377d7 : Constant  Value=-1
  Product_aff36 : Product
  Subtract_aa015 : Sum  Inputs=+-
  Subtract_ad684 : Sum  Inputs=+-
  Blockout_iq_bus_12_5a9dd : Outport
  wires:
  Subtract_aa015/1 -> Subtract_ad684/1
  Constant_-1_377d7/1 -> Product_aff36/1
  Product_aff36/1 -> Add_e4c6d/1
  Add_e4c6d/1 -> Subtract_aa015/1
  State_iq_load_12_82e1a/1 -> Product_aff36/2
  State_iq_line_12_13_b5bd7/1 -> Subtract_aa015/2
  State_iq_line_6_12_a1863/1 -> Add_e4c6d/2
  State_iq_line_12_16_8cacc/1 -> Subtract_ad684/2
  Subtract_ad684/1 -> Blockout_iq_bus_12_5a9dd/1

== system IEEE14_case/AC_1/iq_bus_13_block ==
  note: iq_bus_13 in case14gfl
      | $\mathrm{iq}_{\mathrm{line},6,13}-\mathrm{iq}_{\mathrm{load},13}+\mathrm{iq}_{\mathrm{line},12,13}-\mathrm{iq}_{\mathrm{line},13,14}-\mathrm{iq}_{\mathrm{line},13,17}$
      | Automatically generated on 2025-10-09 21:40:29 .
  State_iq_load_13_3bbcd : Inport
  State_iq_line_6_13_f63e3 : Inport  Port=2
  State_iq_line_12_13_f5a73 : Inport  Port=3
  State_iq_line_13_14_1f5ac : Inport  Port=4
  State_iq_line_13_17_718e0 : Inport  Port=5
  Add_0a89b : Sum
  Add_804f0 : Sum
  Constant_-1_d66d3 : Constant  Value=-1
  Product_12f07 : Product
  Subtract_d7517 : Sum  Inputs=+-
  Subtract_ea7fc : Sum  Inputs=+-
  Blockout_iq_bus_13_89032 : Outport
  wires:
  Add_804f0/1 -> Subtract_d7517/1
  Constant_-1_d66d3/1 -> Product_12f07/1
  Product_12f07/1 -> Add_0a89b/1
  Add_0a89b/1 -> Add_804f0/1
  State_iq_line_6_13_f63e3/1 -> Add_0a89b/2
  State_iq_load_13_3bbcd/1 -> Product_12f07/2
  State_iq_line_12_13_f5a73/1 -> Add_804f0/2
  State_iq_line_13_14_1f5ac/1 -> Subtract_d7517/2
  Subtract_d7517/1 -> Subtract_ea7fc/1
  State_iq_line_13_17_718e0/1 -> Subtract_ea7fc/2
  Subtract_ea7fc/1 -> Blockout_iq_bus_13_89032/1

== system IEEE14_case/AC_1/iq_bus_14_block ==
  note: iq_bus_14 in case14gfl
      | $\mathrm{iq}_{\mathrm{line},9,14}-\mathrm{iq}_{\mathrm{load},14}+\mathrm{iq}_{\mathrm{line},13,14}-\mathrm{iq}_{\mathrm{line},14,18}$
      | Automatically generated on 2025-10-09 21:40:31 .
  State_iq_load_14_41c2f : Inport
  State_iq_line_9_14_48c7f : Inport  Port=2
  State_iq_line_13_14_26ead : Inport  Port=3
  State_iq_line_14_18_e379d : Inport  Port=4
  Add_35714 : Sum
  Add_5250c : Sum
  Constant_-1_a2860 : Constant  Value=-1
  Product_d1f83 : Product
  Subtract_7f4a3 : Sum  Inputs=+-
  Blockout_iq_bus_14_9d2f8 : Outport
  wires:
  Constant_-1_a2860/1 -> Product_d1f83/1
  Product_d1f83/1 -> Add_35714/1
  Add_35714/1 -> Add_5250c/1
  State_iq_load_14_41c2f/1 -> Product_d1f83/2
  State_iq_line_9_14_48c7f/1 -> Add_35714/2
  State_iq_line_14_18_e379d/1 -> Subtract_7f4a3/2
  State_iq_line_13_14_26ead/1 -> Add_5250c/2
  Add_5250c/1 -> Subtract_7f4a3/1
  Subtract_7f4a3/1 -> Blockout_iq_bus_14_9d2f8/1

== system IEEE14_case/AC_1/iq_bus_15_block ==
  note: iq_bus_15 in case14gfl
      | $\mathrm{iq}_{\mathrm{GFL},15}+\mathrm{iq}_{\mathrm{line},11,15}$
      | Automatically generated on 2025-10-09 21:40:34 .
  Input_iq_GFL_15_581cf : Inport
  State_iq_line_11_15_dae91 : Inport  Port=2
  Add_adc01 : Sum
  Blockout_iq_bus_15_665d9 : Outport
  wires:
  State_iq_line_11_15_dae91/1 -> Add_adc01/2
  Input_iq_GFL_15_581cf/1 -> Add_adc01/1
  Add_adc01/1 -> Blockout_iq_bus_15_665d9/1

== system IEEE14_case/AC_1/iq_bus_16_block ==
  note: iq_bus_16 in case14gfl
      | $\mathrm{iq}_{\mathrm{GFL},16}+\mathrm{iq}_{\mathrm{line},12,16}$
      | Automatically generated on 2025-10-09 21:40:36 .
  Input_iq_GFL_16_66c6c : Inport
  State_iq_line_12_16_2996d : Inport  Port=2
  Add_3fe44 : Sum
  Blockout_iq_bus_16_71499 : Outport
  wires:
  State_iq_line_12_16_2996d/1 -> Add_3fe44/2
  Input_iq_GFL_16_66c6c/1 -> Add_3fe44/1
  Add_3fe44/1 -> Blockout_iq_bus_16_71499/1

== system IEEE14_case/AC_1/iq_bus_17_block ==
  note: iq_bus_17 in case14gfl
      | $\mathrm{iq}_{\mathrm{GFL},17}+\mathrm{iq}_{\mathrm{line},13,17}$
      | Automatically generated on 2025-10-09 21:40:39 .
  Input_iq_GFL_17_ce0cb : Inport
  State_iq_line_13_17_ac3bf : Inport  Port=2
  Add_b0f21 : Sum
  Blockout_iq_bus_17_2a23f : Outport
  wires:
  State_iq_line_13_17_ac3bf/1 -> Add_b0f21/2
  Input_iq_GFL_17_ce0cb/1 -> Add_b0f21/1
  Add_b0f21/1 -> Blockout_iq_bus_17_2a23f/1

== system IEEE14_case/AC_1/iq_bus_18_block ==
  note: iq_bus_18 in case14gfl
      | $\mathrm{iq}_{\mathrm{GFL},18}+\mathrm{iq}_{\mathrm{line},14,18}$
      | Automatically generated on 2025-10-09 21:40:42 .
  Input_iq_GFL_18_ec44c : Inport
  State_iq_line_14_18_2108f : Inport  Port=2
  Add_558e8 : Sum
  Blockout_iq_bus_18_97ded : Outport
  wires:
  State_iq_line_14_18_2108f/1 -> Add_558e8/2
  Input_iq_GFL_18_ec44c/1 -> Add_558e8/1
  Add_558e8/1 -> Blockout_iq_bus_18_97ded/1

== system IEEE14_case/AC_1/iq_bus_1_block ==
  note: iq_bus_1 in case14gfl
      | $\mathrm{iq}_{\mathrm{SG},D,1}-\mathrm{iq}_{\mathrm{line},1,2}-\mathrm{iq}_{\mathrm{line},1,5}$
      | Automatically generated on 2025-10-09 21:40:04 .
  Input_iq_SG_D_1_56ece : Inport
  State_iq_line_1_2_a608a : Inport  Port=2
  State_iq_line_1_5_234de : Inport  Port=3
  Subtract_4862a : Sum  Inputs=+-
  Subtract_b07ed : Sum  Inputs=+-
  Blockout_iq_bus_1_352cb : Outport
  wires:
  Subtract_b07ed/1 -> Blockout_iq_bus_1_352cb/1
  Input_iq_SG_D_1_56ece/1 -> Subtract_4862a/1
  State_iq_line_1_2_a608a/1 -> Subtract_4862a/2
  Subtract_4862a/1 -> Subtract_b07ed/1
  State_iq_line_1_5_234de/1 -> Subtract_b07ed/2

== system IEEE14_case/AC_1/iq_bus_2_block ==
  note: iq_bus_2 in case14gfl
      | $\mathrm{iq}_{\mathrm{SG},D,2}-\mathrm{iq}_{\mathrm{load},2}+\mathrm{iq}_{\mathrm{line},1,2}-\mathrm{iq}_{\mathrm{line},2,3}-\mathrm{iq}_{\mathrm{line},2,4}-\mathrm{iq}_{\mathrm{line},2,5}$
      | Automatically generated on 2025-10-09 21:40:07 .
  Input_iq_SG_D_2_8fd05 : Inport
  State_iq_load_2_0a4eb : Inport  Port=2
  State_iq_line_1_2_2f4d7 : Inport  Port=3
  State_iq_line_2_3_ceafd : Inport  Port=4
  State_iq_line_2_4_78218 : Inport  Port=5
  State_iq_line_2_5_fb0c4 : Inport  Port=6
  Add_02fdd : Sum
  Subtract_4d2d3 : Sum  Inputs=+-
  Subtract_56a8e : Sum  Inputs=+-
  Subtract_d7149 : Sum  Inputs=+-
  Subtract_ffa0c : Sum  Inputs=+-
  Blockout_iq_bus_2_d0264 : Outport
  wires:
  Subtract_4d2d3/1 -> Subtract_d7149/1
  Input_iq_SG_D_2_8fd05/1 -> Subtract_56a8e/1
  Subtract_56a8e/1 -> Add_02fdd/1
  State_iq_line_1_2_2f4d7/1 -> Add_02fdd/2
  State_iq_load_2_0a4eb/1 -> Subtract_56a8e/2
  Add_02fdd/1 -> Subtract_4d2d3/1
  State_iq_line_2_4_78218/1 -> Subtract_d7149/2
  State_iq_line_2_3_ceafd/1 -> Subtract_4d2d3/2
  Subtract_d7149/1 -> Subtract_ffa0c/1
  State_iq_line_2_5_fb0c4/1 -> Subtract_ffa0c/2
  Subtract_ffa0c/1 -> Blockout_iq_bus_2_d0264/1

== system IEEE14_case/AC_1/iq_bus_3_block ==
  note: iq_bus_3 in case14gfl
      | $\mathrm{iq}_{\mathrm{SG},D,3}-\mathrm{iq}_{\mathrm{load},3}+\mathrm{iq}_{\mathrm{line},2,3}-\mathrm{iq}_{\mathrm{line},3,4}$
      | Automatically generated on 2025-10-09 21:40:09 .
  Input_iq_SG_D_3_f2caf : Inport
  State_iq_load_3_1a588 : Inport  Port=2
  State_iq_line_2_3_b53b7 : Inport  Port=3
  State_iq_line_3_4_658ee : Inport  Port=4
  Add_5fb9d : Sum
  Subtract_6f6d5 : Sum  Inputs=+-
  Subtract_f19d4 : Sum  Inputs=+-
  Blockout_iq_bus_3_60c7d : Outport
  wires:
  Add_5fb9d/1 -> Subtract_f19d4/1
  State_iq_line_2_3_b53b7/1 -> Add_5fb9d/2
  Subtract_6f6d5/1 -> Add_5fb9d/1
  Input_iq_SG_D_3_f2caf/1 -> Subtract_6f6d5/1
  State_iq_load_3_1a588/1 -> Subtract_6f6d5/2
  State_iq_line_3_4_658ee/1 -> Subtract_f19d4/2
  Subtract_f19d4/1 -> Blockout_iq_bus_3_60c7d/1

== system IEEE14_case/AC_1/iq_bus_4_block ==
  note: iq_bus_4 in case14gfl
      | $\mathrm{iq}_{\mathrm{line},2,4}-\mathrm{iq}_{\mathrm{load},4}+\mathrm{iq}_{\mathrm{line},3,4}-\mathrm{iq}_{\mathrm{line},4,5}-\mathrm{iq}_{\mathrm{line},4,7}-\mathrm{iq}_{\mathrm{line},4,9}$
      | Automatically generated on 2025-10-09 21:40:11 .
  State_iq_load_4_ce024 : Inport
  State_iq_line_2_4_9abf1 : Inport  Port=2
  State_iq_line_3_4_962a3 : Inport  Port=3
  State_iq_line_4_5_4a221 : Inport  Port=4
  State_iq_line_4_7_17bcc : Inport  Port=5
  State_iq_line_4_9_e8dca : Inport  Port=6
  Add_57cd3 : Sum
  Add_a524b : Sum
  Constant_-1_8c9ab : Constant  Value=-1
  Product_0a559 : Product
  Subtract_55296 : Sum  Inputs=+-
  Subtract_9f712 : Sum  Inputs=+-
  Subtract_ce063 : Sum  Inputs=+-
  Blockout_iq_bus_4_8bc6d : Outport
  wires:
  State_iq_line_3_4_962a3/1 -> Add_57cd3/2
  State_iq_line_2_4_9abf1/1 -> Add_a524b/2
  Constant_-1_8c9ab/1 -> Product_0a559/1
  State_iq_load_4_ce024/1 -> Product_0a559/2
  Product_0a559/1 -> Add_a524b/1
  Add_a524b/1 -> Add_57cd3/1
  Subtract_55296/1 -> Subtract_9f712/1
  Add_57cd3/1 -> Subtract_ce063/1
  State_iq_line_4_5_4a221/1 -> Subtract_ce063/2
  Subtract_ce063/1 -> Subtract_55296/1
  State_iq_line_4_7_17bcc/1 -> Subtract_55296/2
  Subtract_9f712/1 -> Blockout_iq_bus_4_8bc6d/1
  State_iq_line_4_9_e8dca/1 -> Subtract_9f712/2

== system IEEE14_case/AC_1/iq_bus_5_block ==
  note: iq_bus_5 in case14gfl
      | $\mathrm{iq}_{\mathrm{line},1,5}-\mathrm{iq}_{\mathrm{load},5}+\mathrm{iq}_{\mathrm{line},2,5}+\mathrm{iq}_{\mathrm{line},4,5}-\mathrm{iq}_{\mathrm{line},5,6}$
      | Automatically generated on 2025-10-09 21:40:13 .
  State_iq_load_5_72501 : Inport
  State_iq_line_1_5_5a6f8 : Inport  Port=2
  State_iq_line_2_5_08804 : Inport  Port=3
  State_iq_line_4_5_98539 : Inport  Port=4
  State_iq_line_5_6_789df : Inport  Port=5
  Add_407f8 : Sum
  Add_8334a : Sum
  Add_e4e2c : Sum
  Constant_-1_4cb9c : Constant  Value=-1
  Product_3bc14 : Product
  Subtract_0629e : Sum  Inputs=+-
  Blockout_iq_bus_5_f0651 : Outport
  wires:
  Add_e4e2c/1 -> Subtract_0629e/1
  Add_8334a/1 -> Add_e4e2c/1
  Constant_-1_4cb9c/1 -> Product_3bc14/1
  Product_3bc14/1 -> Add_407f8/1
  Add_407f8/1 -> Add_8334a/1
  State_iq_line_1_5_5a6f8/1 -> Add_407f8/2
  State_iq_load_5_72501/1 -> Product_3bc14/2
  State_iq_line_2_5_08804/1 -> Add_8334a/2
  State_iq_line_4_5_98539/1 -> Add_e4e2c/2
  State_iq_line_5_6_789df/1 -> Subtract_0629e/2
  Subtract_0629e/1 -> Blockout_iq_bus_5_f0651/1
